simulink library "marine_lib_sys"  (R2024a)
settings: Solver=VariableStepAuto  StartTime=0.0  StopTime=10.0  RelTol=1e-3
undefined symbols (not defined in the file): ss_x, ss_yaw
settings Model: Creator=luka  LastModifiedBy=luka

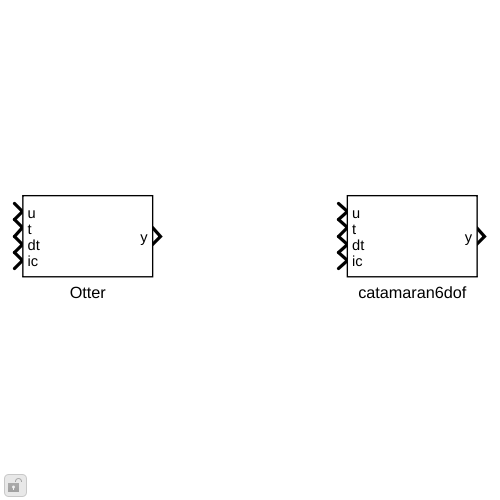
[thumbnail: Simulink's stored preview of the top-level diagram]
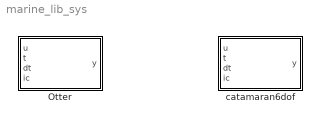
== system marine_lib_sys ==
  Otter : Subsystem  Tag=system;__cs_slx_sys;__cs_comptype:sys;__cs_compimpl:slx;  mask{payload_mass=0, payload_location=[0,0, 0], current_speed=0, current_direction=0, out_gain=1, iid__=[0], pid__=[79 116 116 101 114 58 109 97 114 105 110 101 95 108 105 98], context_path=, params=[], params_struct_name=}
      mask prompts: payload_mass "Payload mass"; payload_location "Payload location"; current_speed "Current speed"; current_direction "Current direction"
  catamaran6dof : Subsystem  Tag=__cs_comptype:sys;__cs_compimpl:slx;  mask{iid__=[0], pid__=[99 97 116 97 109 97 114 97 110 54 100 111 102 58 109 97 114 105 110 101 95 108 105 98], context_path=, params=[], params_struct_name=}

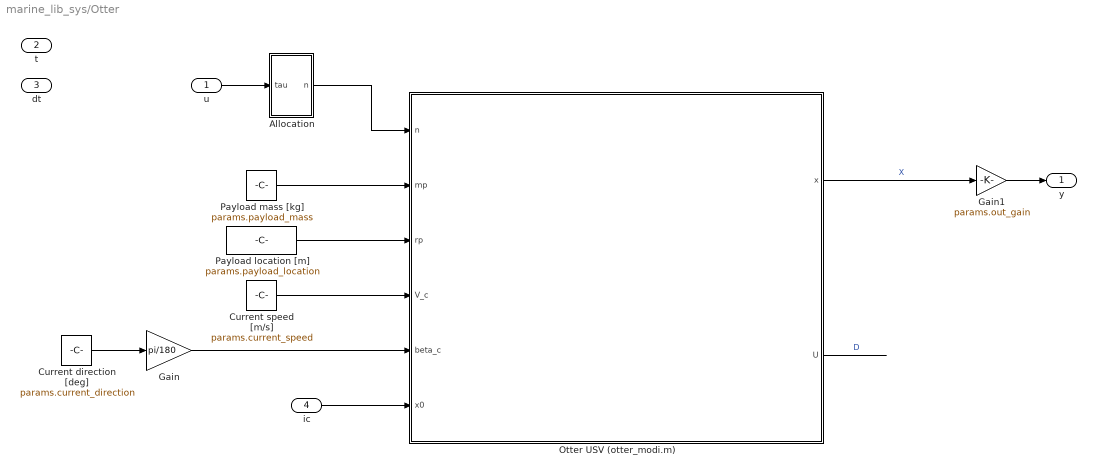
== system marine_lib_sys/Otter ==
  u : Inport  PortDimensions=2
  t : Inport  Port=2
  dt : Inport  Port=3
  ic : Inport  Port=4
  Allocation : Subsystem
  Current direction [deg] : Constant  Value=params.current_direction
  Current speed [m/s] : Constant  Value=params.current_speed
  Gain : Gain  Gain=pi/180
  Gain1 : Gain  Gain=params.out_gain
  "Otter USV (otter_modi.m) " : Subsystem  AncestorBlock=mssSimulink/Marine craft models/Otter USV (otter.m)
      settings: LibrarySourceBlock=mssSimulink/Marine craft models/Otter USV (otter.m)
      mask Display: image('otter.jpg'); % Use "Edit Image" on toolstrip to change.
  Payload location [m] : Constant  Value=params.payload_location  VectorParams1D=off
  Payload mass [kg] : Constant  Value=params.payload_mass
  y : Outport  PortDimensions=12
  wires:
  Gain1/1 -> y/1
  Payload mass [kg]/1 -> "Otter USV (otter_modi.m) "/2(mp)
  u/1 -> Allocation/1(tau)
  Gain/1 -> "Otter USV (otter_modi.m) "/5(beta_c)
  Payload location [m]/1 -> "Otter USV (otter_modi.m) "/3(rp)
  ic/1 -> "Otter USV (otter_modi.m) "/6(x0)
  "Otter USV (otter_modi.m) "/1(x) -> Gain1/1  "X"
  Current speed [m/s]/1 -> "Otter USV (otter_modi.m) "/4(V_c)
  Allocation/1(n) -> "Otter USV (otter_modi.m) "/1(n)
  "Otter USV (otter_modi.m) "/2(U) -> ?  "D"
  Current direction [deg]/1 -> Gain/1

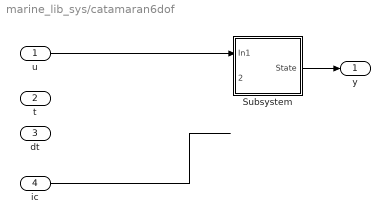
== system marine_lib_sys/catamaran6dof ==
  u : Inport  PortDimensions=2
  t : Inport  Port=2
  dt : Inport  Port=3
  ic : Inport  Port=4
  Subsystem : Subsystem
  y : Outport  PortDimensions=6
  wires:
  u/1 -> Subsystem/1(In1)
  Subsystem/1(State) -> y/1
  ic/1 -> ?

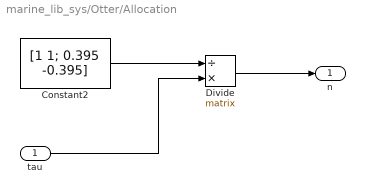
== system marine_lib_sys/Otter/Allocation ==
  tau : Inport
  Constant2 : Constant  Value=[1 1; 0.395 -0.395]
  Divide : Product  Inputs=/*  Multiplication=Matrix(*)
  n : Outport
  wires:
  tau/1 -> Divide/2
  Divide/1 -> n/1
  Constant2/1 -> Divide/1

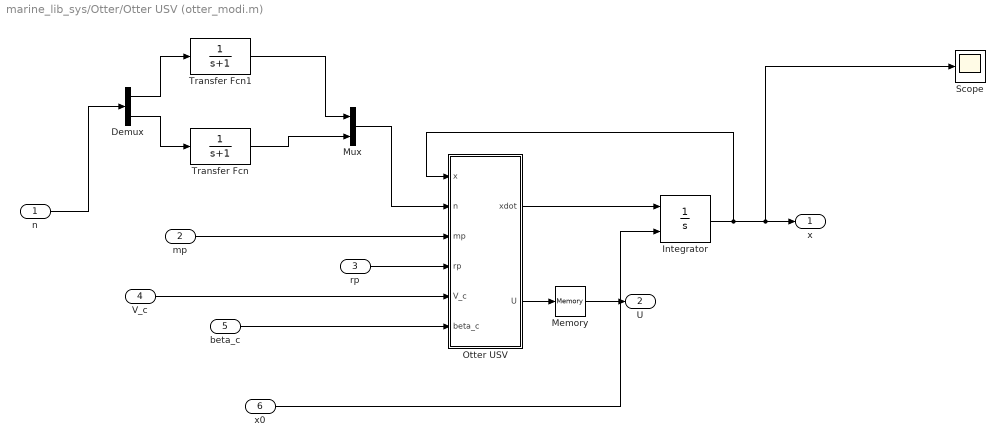
== system marine_lib_sys/Otter/Otter USV (otter_modi.m)  ==
  n : Inport
  mp : Inport  Port=2
  rp : Inport  Port=3
  V_c : Inport  Port=4
  beta_c : Inport  Port=5
  x0 : Inport  Port=6
  Demux : Demux  Outputs=2
  Integrator : Integrator  InitialConditionSource=external  InitialCondition=[1 1]  UpperSaturationLimit=10  LowerSaturationLimit=-10
  Memory : Memory
  Mux : Mux  Inputs=2
  Otter USV : MATLAB Function  TreatAsAtomicUnit=on
  Scope : Scope
  Transfer Fcn : TransferFcn  Denominator=[1 1]
  Transfer Fcn1 : TransferFcn  Denominator=[1 1]
  x : Outport
  U : Outport  Port=2
  wires:
  Integrator/1 -> x/1, Scope/1, Otter USV/1(x)
  Mux/1 -> Otter USV/2(n)
  n/1 -> Demux/1
  Memory/1 -> U/1
  x0/1 -> Integrator/2
  rp/1 -> Otter USV/4(rp)
  beta_c/1 -> Otter USV/6(beta_c)
  Otter USV/1(xdot) -> Integrator/1
  mp/1 -> Otter USV/3(mp)
  Otter USV/2(U) -> Memory/1
  V_c/1 -> Otter USV/5(V_c)
  Demux/1 -> Transfer Fcn1/1
  Demux/2 -> Transfer Fcn/1
  Transfer Fcn/1 -> Mux/2
  Transfer Fcn1/1 -> Mux/1

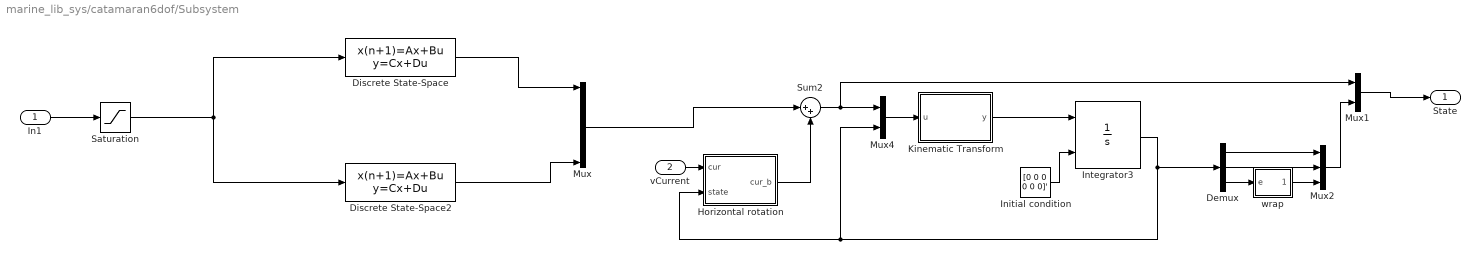
== system marine_lib_sys/catamaran6dof/Subsystem ==
  In1 : Inport
  vCurrent : Inport  Port=2
  Demux : Demux  Outputs=3
  Discrete State-Space : DiscreteStateSpace  A=ss_x.A  B=ss_x.B  C=ss_x.C  D=ss_x.D  SampleTime=ss_x.Ts
  Discrete State-Space2 : DiscreteStateSpace  A=ss_yaw.A  B=ss_yaw.B  C=ss_yaw.C  D=ss_yaw.D  SampleTime=ss_yaw.Ts
  Horizontal rotation : MATLAB Function  TreatAsAtomicUnit=on
  Initial condition : Constant  Value=[0 0 0 0 0 0]'
  Integrator3 : Integrator  InitialConditionSource=external
  Kinematic Transform : MATLAB Function  TreatAsAtomicUnit=on
  Mux : Mux  Inputs=6
  Mux1 : Mux  Inputs=2
  Mux2 : Mux  Inputs=3
  Mux4 : Mux  Inputs=2
  Saturation : Saturate  UpperLimit=1  LowerLimit=-1
  Sum2 : Sum  Inputs=|++
  wrap : MATLAB Function  TreatAsAtomicUnit=on
  State : Outport
  wires:
  In1/1 -> Saturation/1
  Discrete State-Space2/1 -> Mux/6
  Kinematic Transform/1(y) -> Integrator3/1
  Initial condition/1 -> Integrator3/2
  Sum2/1 -> Mux1/1, Mux4/1
  vCurrent/1 -> Horizontal rotation/1(cur)
  Mux4/1 -> Kinematic Transform/1(u)
  Integrator3/1 -> Demux/1, Horizontal rotation/2(state), Mux4/2
  Mux/1 -> Sum2/1
  Horizontal rotation/1(cur_b) -> Sum2/2
  Mux1/1 -> State/1
  Discrete State-Space/1 -> Mux/1
  Demux/3 -> wrap/1(e)
  wrap/1(ew) -> Mux2/3
  Demux/1 -> Mux2/1
  Demux/2 -> Mux2/2
  Mux2/1 -> Mux1/2
  Saturation/1 -> Discrete State-Space2/1, Discrete State-Space/1

== matlab function marine_lib_sys/catamaran6dof/Subsystem/Horizontal rotation ==
  data: cur input; cur_b output; state input
function cur_b = fcn(cur, state)
cur_b = zeros(6,1);
Psi = state(6,1);
R_z_psi = [cos(Psi) sin(Psi); -sin(Psi) cos(Psi)];

cur_ne_b = R_z_psi*cur;
cur_b(1) = cur_ne_b(1);
cur_b(2) = cur_ne_b(2);

== matlab function marine_lib_sys/Otter/Otter USV (otter_modi.m) /Otter USV ==
  settings: updateMethod=DISCRETE
  data: x input; n input; xdot output; mp input; rp input; V_c input; beta_c input; U output
function [xdot, U] = fcn(x,n,mp,rp,V_c,beta_c)

[xdot,U] = otter(x,n,mp,rp,V_c,beta_c);

end

== matlab function marine_lib_sys/catamaran6dof/Subsystem/Kinematic Transform ==
  data: u input; y output
function y = fcn(u)
%#codegen
if (length(u)<12) 
    y = zeros(12,1);
    return;
end

input = u;
% Read inputs
u = input(1,1);
v = input(2,1);
w = input(3,1);
p = input(4,1);
q = input(5,1);
r = input(6,1);

%x = input(7,1);
%y = input(8,1);
%z = input(9,1);
phi = input(10,1);
theta = input(11,1);
Psi = input(12,1);

DOF6 = 1; % Select degrees of freedom

tmp1 = []; tmp2 = [];

if DOF6 == 1
    
    % Rotation matrix
    R_x_phi = [1 0 0; 0 cos(phi) sin(phi); 0 -sin(phi) cos(phi)];
    R_y_theta = [cos(theta) 0 -sin(theta); 0 1 0; sin(theta) 0 cos(theta)];% Provjeri matrice
    R_z_psi = [cos(Psi) sin(Psi) 0; -sin(Psi) cos(Psi) 0; 0 0 1];
    
    % Linear velocity transform
    J1 = R_z_psi.'*R_y_theta.'*R_x_phi.';
    
    % Angular velocity transform    
    tmp1 = R_x_phi(:,2);
    tmp1 = [0 0 0; tmp1.'; 0 0 0].';
    
    tmp2 = R_x_phi*R_y_theta;
    tmp2 = tmp2(:,3);
    tmp2 = [0 0 0; 0 0 0; tmp2.'].';
    
    J2 = inv(diag([1 0 0])+tmp1+tmp2);
    
elseif DOF6 == 0
    
    % Rotation matrix
    R_x_phi = eye(3);
    R_y_theta = eye(3);
    R_z_psi = [cos(Psi) sin(Psi) 0; -sin(Psi) cos(Psi) 0; 0 0 1]; % Provjeri matrice
    
    % Linear velocity transform
    J1 = R_z_psi.'*R_y_theta.'*R_x_phi.';
    
    % Angular velocity transform 
    tmp1 = R_x_phi(:,2);
    tmp1 = [0 0 0; tmp1.'; 0 0 0].';
    
    tmp2 = R_x_phi*R_y_theta;
    tmp2 = tmp2(:,3);
    tmp2 = [0 0 0; 0 0 0; tmp2.'].';
    
    J2 = inv(diag([1 0 0])+tmp1+tmp2);
    
end

eta1 = J1*[u v w].';
eta2 = J2*[p q r].';


y = [eta1.' eta2.'].';

== matlab function marine_lib_sys/catamaran6dof/Subsystem/wrap ==
  data: e input; ew output
function ew = wrap(e)

ew = mod(e, 2*pi);

if ew > pi
   ew = -2*pi + ew;
elseif ew <= -pi 
   ew = 2*pi + ew;
end
